simulink subsystem "mfc_F_est_disc"  (R2026a)
settings: Solver=FixedStepDiscrete  FixedStep=Ts
values from neighbouring files (symbols this model uses):
  Ts = 0.01    [build_mfc_lib.m]
undefined symbols (not defined in the file or in its folder): DiscIntNeverNeededParam
settings Model: Creator=devinbellll  LastModifiedBy=devinbellll

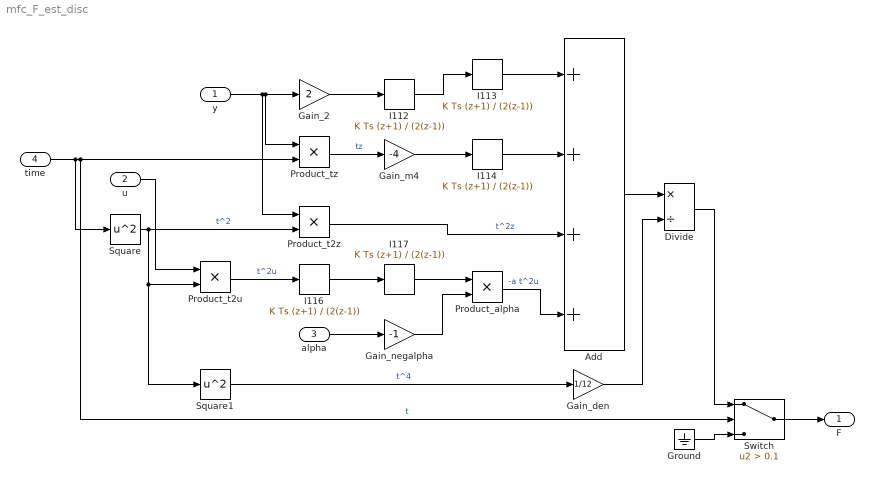
== system mfc_F_est_disc ==
  y : Inport
  u : Inport  Port=2
  alpha : Inport  Port=3
  time : Inport  Port=4
  Add : Sum  Inputs=++++
  Divide : Product  Inputs=*/
  Gain_2 : Gain  Gain=2
  Gain_den : Gain  Gain=1/12
  Gain_m4 : Gain  Gain=-4
  Gain_negalpha : Gain  Gain=-1
  Ground : Ground
  I{112..114,116..117} (5 alike) : DiscreteIntegrator  IntegratorMethod=Integration: Trapezoidal  SampleTime=Ts  ICPrevOutput=DiscIntNeverNeededParam  ICPrevScaledInput=DiscIntNeverNeededParam
  Product_alpha : Product
  Product_t2u : Product
  Product_t2z : Product
  Product_tz : Product
  Square : Math  Operator=square
  Square1 : Math  Operator=square
  Switch : Switch  Criteria=u2 > Threshold  Threshold=0.1  SaturateOnIntegerOverflow=off  InputSameDT=off
  F : Outport
  wires:
  Divide/1 -> Switch/1
  Gain_den/1 -> Divide/2
  Add/1 -> Divide/1
  Product_alpha/1 -> Add/4  "-a t^2u"
  Gain_negalpha/1 -> Product_alpha/2
  I117/1 -> Product_alpha/1
  Ground/1 -> Switch/3
  Gain_m4/1 -> I114/1
  Product_t2z/1 -> Add/3  "t^2z"
  I113/1 -> Add/1
  Product_tz/1 -> Gain_m4/1  "tz"
  Gain_2/1 -> I112/1
  Square1/1 -> Gain_den/1  "t^4"
  Product_t2u/1 -> I116/1  "t^2u"
  I114/1 -> Add/2
  I112/1 -> I113/1
  y/1 -> Gain_2/1, Product_tz/1, Product_t2z/1
  Square/1 -> Square1/1, Product_t2u/2, Product_t2z/2  "t^2"
  u/1 -> Product_t2u/1
  alpha/1 -> Gain_negalpha/1
  I116/1 -> I117/1
  Switch/1 -> F/1
  time/1 -> Product_tz/2, Switch/2, Square/1  "t"
